simulink model "mech_robot"  (Simulink 6.0)
settings: Solver=ode15s  StartTime=0.0  StopTime=1  RelTol=1e-3  AbsTol=1e-4
PreLoadFcn:
  | load mech_robot_images;mech_robot_data;
undefined symbols (not defined in the file or in its folder): Actuator, rad, s
libraries: mblibv1 x88, mech_robot_vrlib x1
(part 1 of 3)
settings Model: Creator=gwood  LastModifiedBy=batserve  ExtModeAutoUpdateStatusClock=off  ProdHWDeviceType=Specified
settings DataIOCC: SignalLoggingName=sigsOut  OutputTimes=0:0.02:1
settings DebuggingCC: AlgebraicLoopMsg=none  CheckExecutionContextPreStartOutputMsg=on  CheckExecutionContextRuntimeOutputMsg=on  SolverPrmCheckMsg=none  UnconnectedInputMsg=none  UnconnectedOutputMsg=none  UnconnectedLineMsg=none
settings HardwareCC: ProdBitPerShort=32  ProdBitPerInt=16  ProdHWDeviceType=Specified  TargetUnknown=on

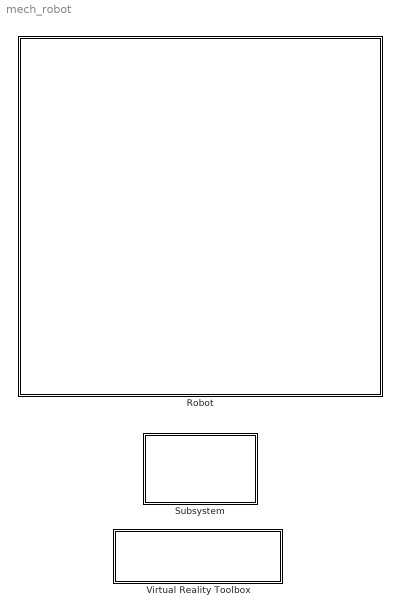
== system mech_robot ==
  Robot : Subsystem
      mask Display: image(robot);
  Subsystem : Subsystem
      mask Display: disp('Model Information');
  Virtual Reality Toolbox : Subsystem
      settings: AttributesFormatString=\n  OpenFcn=mech_OpenVrWorld(gcs,'mech_robot_vrlib')
      mask Type: Double-click open
      mask Display: disp(sprintf('Double-click to open\nVirtual Reality Toolbox viewer'))

== system mech_robot/Robot ==
  Joint Angles : Scope
  Link 1 : Subsystem  Orientation=up
      mask Display: image(rbody1)
  Link 2 : Subsystem
      mask Display: image(rbody2);
  Link3 : Subsystem  Orientation=up
      mask Display: image(rbody3);
  Link4 : Subsystem  Orientation=up
      mask Display: image(rbody4);
  Link5 : Subsystem  Orientation=up
      mask Display: image(rbody5);
  Link6 : Subsystem  Orientation=up
      mask Display: image(rdrill);
  Mux : Mux  Inputs=6
  Robot base : Subsystem  Orientation=up
      mask Display: image(rbase);
  wires:
  [Body1] -> Mux/1
  [Body2] -> Mux/2
  [Body3] -> Mux/3
  [Body4] -> Mux/4
  [Body5] -> Mux/5
  [Body6] -> Mux/6
  Mux/1 -> Joint Angles/1
  connections:
  Robot base/RConn1 -- Link 1/LConn1
  Link 1/RConn1 -- Link 2/LConn1
  Link 2/RConn1 -- Link3/LConn1
  Link3/RConn1 -- Link4/LConn1
  Link4/RConn1 -- Link5/LConn1
  Link5/RConn1 -- Link6/LConn1

== system mech_robot/Subsystem ==
  note: This model is a detailed dynamic model of the Siemens Manutec r3 robot. All of the important physical effects are
      | included, notably: the multibody dynamics, Coulomb friction, elasticity and damping in the gearboxes, the dynamics
      | of the motors including the current controller and the tachogenerators, and the cascade controllers. All of the parameters
      | of this model were obtained by experiment and can be found in the following paper. This model is used as a demanding
      | benchmark to test the simulation capabilites of robot simulation packages.
  note: "The Manutec r3 Benchmark Models for Dynamic Simulation of Robots", DLR FF-DR-ER, Technical Report TR T101-93,
      | March 1993.
  note: Paper available at: www.citeseer.com

== system mech_robot/Virtual Reality Toolbox ==
  VRAnimation : mech_robot_vrlib/mech_robot_arm_vr

== system mech_robot/Robot/Link 1 ==
  Body1 : mblibv1/Bodies/Body  Tag=Factory generic  Description=Mechanical Blockset  Orientation=up  PhysicalDomain=mechanical  SubClassName=Unknown  LeftPortType=workingframe  RightPortType=workingframe  LConnTagsString=CS1  RConnTagsString=CS2  DialogClass=MechanicalBodyBlock  Mass=0  MassUnits=kg  InertiaUnits=kg*m^2  Inertia=diag([0 1.16 0])  Shape=Cylinder  ShapeDims=[1 1]  ShapeUnits=m  ShapeUse=false  Density=1  DensityUnits=kg/m^3  DensityUse=false  CG=Left$CG$[0 -0.1750+0.25/2 0]$WORLD$WORLD$m$[0 0 0]$Euler X-Y-Z$deg$WORLD$false  WorkingFrames=Left$CS1$[0 -0.1750 0]$WORLD$WORLD$m$[0 0 0]$Euler X-Y-Z$deg$WORLD$true#Right$CS2$[0.075 0 0]$WORLD$WORLD$m$[0 0 0]$Euler X-Y-Z$deg$WORLD$true#Right$CS3$[-0.075 -0.1750 0.1]$CG$CG$m$[0 0 0]$Euler X-Y-Z$deg$WORLD$false#Right$CS4$[0.075 -0.1750 0.1]$CG$CG$m$[0 0 0]$Euler X-Y-Z$deg$WORLD$false#Right$CS5$[0.075 -0.1750 -0.1]$CG$CG$m$[0 0 0]$Euler X-Y-Z$deg$WORLD$false#Right$CS6$[-0.075 -0.1750 -0.1]$CG$CG$m$[0 0 0]$Euler X-Y-Z$deg$WORLD$false#Right$CS7$[-0.075 0.075 0.1]$CG$CG$m$[0 0 0]$Euler X-Y-Z$deg$WORLD$false#Right$CS8$[0.075 0.075 0.1]$CG$CG$m$[0 0 0]$Euler X-Y-Z$deg$WORLD$false#Right$CS9$[0.075 0.075 -0.1]$CG$CG$m$[0 0 0]$Euler X-Y-Z$deg$WORLD$false#Right$CS10$[-0.075 0.075 -0.1]$CG$CG$m$[0 0 0]$Euler X-Y-Z$deg$WORLD$false
  Drive1 : Subsystem  Orientation=up  mask{q0=-1, Actuator=Actuator{1}}
      mask prompts: q0 "Initial angle (rad)"; Actuator "Actuator data structure"
      settings: AttributesFormatString=\n
      mask Display: plot(-80,-80,80,80,[0,9,18,24,29,30,29,24,18,9,0,-9,-18,-24,-29,-30,-29,-24,-18,-9,0],[30,29,24,18,9,0,-9,-18,-24,-29,-30,-29,-24,-18,-9,0,9,18,24,29,30],[-29,-35,-35,-29],[-8,-8,8,8],[29,35,35,29],[-8,-8,8,8],[-35,-55],[0,0],[35,55],[0,0],[-78,-50,-50,-49,-45,-39,-33,-26,-21,-18,-17,-19,-22,-22,-26,-27,-25,-22,-16,-9,-3,2,6,6,4,1,1,-3,-4,-2,2,7,14,20,26,29,30,28,24,24,21,20,21,25,31,37,44,49,50,50,50,78]*.7,[58,58,57.2,49.2,42.8,38.8,38,39.6,44.4,51.6,59.6,67.6,72.4,72.4,65.2,57.2,49.2,42.8,38.8,38,39.6,44.4,51.6,59.6,67.6,72.4,72.4,65.2,57.2,49.2,42.8,38.8,38,39.6,44.4,51.6,59.6,67.6,72.4,72.4,65.2,57.2,49.2,42.8,38.8,38,39.6,44.4,51.6,58,58,58]*.6+15 );
  Trajectory 1 : Subsystem
  Follower : PMIOPort  Orientation=down  Port=1  Side=Right
  Base : PMIOPort  Orientation=up  Port=2  Side=Left
  wires:
  Trajectory 1/1(Acceleration1) -> Drive1/1(Acceleration)
  connections:
  Drive1/RConn1 -- Body1/LConn1
  Follower/RConn1 -- Body1/RConn1
  Base/RConn1 -- Drive1/LConn1

== system mech_robot/Robot/Link 2 ==
  Body2 : mblibv1/Bodies/Body  Tag=Factory generic  Description=Mechanical Blockset  Orientation=up  PhysicalDomain=mechanical  SubClassName=Unknown  LeftPortType=workingframe  RightPortType=workingframe  LConnTagsString=CS1  RConnTagsString=CS2  DialogClass=MechanicalBodyBlock  Mass=56.5  MassUnits=kg  InertiaUnits=kg*m^2  Inertia=[2.58 -0.46 0;-0.46 0.64 0;0 0 2.73]  Shape=Cylinder  ShapeDims=[1 1]  ShapeUnits=m  ShapeUse=false  Density=1  DensityUnits=kg/m^3  DensityUse=false  CG=Left$CG$[0.172 0.205 0]$WORLD$WORLD$m$[0 0 0]$Euler X-Y-Z$deg$WORLD$false  WorkingFrames=Left$CS1$[0.075 0 0]$WORLD$WORLD$m$[0 0 0]$Euler X-Y-Z$deg$WORLD$true#Right$CS2$[0.075 0.5 0]$WORLD$WORLD$m$[0 0 0]$Euler X-Y-Z$deg$WORLD$true#Right$CS3$[0.075 -0.1 0.1]$WORLD$WORLD$m$[0 0 0]$Euler X-Y-Z$deg$WORLD$false#Right$CS4$[0.075 0.6 0.1]$WORLD$WORLD$m$[0 0 0]$Euler X-Y-Z$deg$WORLD$false#Right$CS5$[0.075 0.6 -0.1]$WORLD$WORLD$m$[0 0 0]$Euler X-Y-Z$deg$WORLD$false#Right$CS6$[0.075 -0.1 -0.1]$WORLD$WORLD$m$[0 0 0]$Euler X-Y-Z$deg$WORLD$false#Right$CS7$[0.225 -0.1 -0.1]$WORLD$WORLD$m$[0 0 0]$Euler X-Y-Z$deg$WORLD$false#Right$CS8$[0.225 -0.1 0.1]$WORLD$WORLD$m$[0 0 0]$Euler X-Y-Z$deg$WORLD$false#Right$CS9$[0.225 0.6 0.1]$WORLD$WORLD$m$[0 0 0]$Euler X-Y-Z$deg$WORLD$false#Right$CS10$[0.225 0.6 -0.1]$WORLD$WORLD$m$[0 0 0]$Euler X-Y-Z$deg$WORLD$false
  Drive2 : Subsystem  Orientation=up  mask{q0=0.43, Actuator=Actuator{2}}
      mask prompts: q0 "Initial angle (rad)"; Actuator "Actuator data structure"
      mask Display: plot(-80,-80,80,80,[0,9,18,24,29,30,29,24,18,9,0,-9,-18,-24,-29,-30,-29,-24,-18,-9,0],[30,29,24,18,9,0,-9,-18,-24,-29,-30,-29,-24,-18,-9,0,9,18,24,29,30],[-29,-35,-35,-29],[-8,-8,8,8],[29,35,35,29],[-8,-8,8,8],[-35,-55],[0,0],[35,55],[0,0],[-78,-50,-50,-49,-45,-39,-33,-26,-21,-18,-17,-19,-22,-22,-26,-27,-25,-22,-16,-9,-3,2,6,6,4,1,1,-3,-4,-2,2,7,14,20,26,29,30,28,24,24,21,20,21,25,31,37,44,49,50,50,50,78]*.7,[58,58,57.2,49.2,42.8,38.8,38,39.6,44.4,51.6,59.6,67.6,72.4,72.4,65.2,57.2,49.2,42.8,38.8,38,39.6,44.4,51.6,59.6,67.6,72.4,72.4,65.2,57.2,49.2,42.8,38.8,38,39.6,44.4,51.6,59.6,67.6,72.4,72.4,65.2,57.2,49.2,42.8,38.8,38,39.6,44.4,51.6,58,58,58]*.6+15 );
  Subsystem : Subsystem
  Follower : PMIOPort  Orientation=down  Port=1  Side=Right
  Base : PMIOPort  Orientation=up  Port=2  Side=Left
  wires:
  Subsystem/1(Acceleration2) -> Drive2/1(Acceleration)
  connections:
  Follower/RConn1 -- Body2/RConn1
  Base/RConn1 -- Drive2/LConn1
  Drive2/RConn1 -- Body2/LConn1

== system mech_robot/Robot/Link3 ==
  Acceleration3 : Subsystem
  Body3 : mblibv1/Bodies/Body  Tag=Factory generic  Description=Mechanical Blockset  Orientation=up  PhysicalDomain=mechanical  SubClassName=Unknown  LeftPortType=workingframe  RightPortType=workingframe  LConnTagsString=CS1  RConnTagsString=CS2  DialogClass=MechanicalBodyBlock  Mass=26.4  MassUnits=kg  InertiaUnits=kg*m^2  Inertia="[0.279  -0.070  0;-0.070  0.245  0;0  0   0.413]"  Shape=Cylinder  ShapeDims=[1 1]  ShapeUnits=m  ShapeUse=false  Density=1  DensityUnits=kg/m^3  DensityUse=false  CG=Left$CG$[0.064 0.5-0.034 0]$WORLD$WORLD$m$[0 0 0]$Euler X-Y-Z$deg$WORLD$false  WorkingFrames=Left$CS1$[0.075 0.5 0]$WORLD$WORLD$m$[0 0 0]$Euler X-Y-Z$deg$WORLD$true#Right$CS2$[0 0.5+0.075 0]$WORLD$WORLD$m$[0 0 0]$Euler X-Y-Z$deg$WORLD$true#Right$CS3$[-0.075 0.5-0.075 0.075]$WORLD$WORLD$m$[0 0 0]$Euler X-Y-Z$deg$WORLD$false#Right$CS4$[0.075 0.5-0.075 0.075]$WORLD$WORLD$m$[0 0 0]$Euler X-Y-Z$deg$WORLD$false#Right$CS5$[0.075 0.5-0.075 -0.075]$WORLD$WORLD$m$[0 0 0]$Euler X-Y-Z$deg$WORLD$false#Right$CS6$[-0.075 0.5-0.075 -0.075]$WORLD$WORLD$m$[0 0 0]$Euler X-Y-Z$deg$WORLD$false#Right$CS7$[-0.075 0.5+0.075 0.075]$WORLD$WORLD$m$[0 0 0]$Euler X-Y-Z$deg$WORLD$false#Right$CS8$[-0.075 0.5+0.075 -0.075]$WORLD$WORLD$m$[0 0 0]$Euler X-Y-Z$deg$WORLD$false#Right$CS9$[0.075 0.5+0.075 -0.075]$WORLD$WORLD$m$[0 0 0]$Euler X-Y-Z$deg$WORLD$false#Right$CS10$[0.075 0.5+0.075 0.075]$WORLD$WORLD$m$[0 0 0]$Euler X-Y-Z$deg$WORLD$false
  Drive3 : Subsystem  Orientation=up  mask{q0=1.57, Actuator=Actuator{3}}
      mask prompts: q0 "Initial angle (rad)"; Actuator "Actuator data structure"
      mask Display: plot(-80,-80,80,80,[0,9,18,24,29,30,29,24,18,9,0,-9,-18,-24,-29,-30,-29,-24,-18,-9,0],[30,29,24,18,9,0,-9,-18,-24,-29,-30,-29,-24,-18,-9,0,9,18,24,29,30],[-29,-35,-35,-29],[-8,-8,8,8],[29,35,35,29],[-8,-8,8,8],[-35,-55],[0,0],[35,55],[0,0],[-78,-50,-50,-49,-45,-39,-33,-26,-21,-18,-17,-19,-22,-22,-26,-27,-25,-22,-16,-9,-3,2,6,6,4,1,1,-3,-4,-2,2,7,14,20,26,29,30,28,24,24,21,20,21,25,31,37,44,49,50,50,50,78]*.7,[58,58,57.2,49.2,42.8,38.8,38,39.6,44.4,51.6,59.6,67.6,72.4,72.4,65.2,57.2,49.2,42.8,38.8,38,39.6,44.4,51.6,59.6,67.6,72.4,72.4,65.2,57.2,49.2,42.8,38.8,38,39.6,44.4,51.6,59.6,67.6,72.4,72.4,65.2,57.2,49.2,42.8,38.8,38,39.6,44.4,51.6,58,58,58]*.6+15 );
  Follower : PMIOPort  Orientation=down  Port=1  Side=Right
  Base : PMIOPort  Orientation=up  Port=2  Side=Left
  wires:
  Acceleration3/1(Acceleration3) -> Drive3/1(Acceleration)
  connections:
  Drive3/RConn1 -- Body3/LConn1
  Follower/RConn1 -- Body3/RConn1
  Base/RConn1 -- Drive3/LConn1

== system mech_robot/Robot/Link4 ==
  Body4 : mblibv1/Bodies/Body  Tag=Factory generic  Description=Mechanical Blockset  Orientation=up  PhysicalDomain=mechanical  SubClassName=Unknown  LeftPortType=workingframe  RightPortType=workingframe  LConnTagsString=CS1  RConnTagsString=CS2  DialogClass=MechanicalBodyBlock  Mass=28.7  MassUnits=kg  InertiaUnits=kg*m^2  Inertia=[1.67 0 0;0 0.081 0;0 0 1.67]  Shape=Cylinder  ShapeDims=[1 1]  ShapeUnits=m  ShapeUse=false  Density=1  DensityUnits=kg/m^3  DensityUse=false  CG=Left$CG$[0 0.5+0.32 0]$WORLD$WORLD$m$[0 0 0]$Euler X-Y-Z$deg$WORLD$false  WorkingFrames=Left$CS1$[0 0.5+0.075 0]$WORLD$WORLD$m$[0 0 0]$Euler X-Y-Z$deg$WORLD$true#Right$CS2$[0 0.5+0.73 0]$WORLD$WORLD$m$[0 0 0]$Euler X-Y-Z$deg$WORLD$true#Right$CS3$[-0.05 0.5+0.075 -0.05]$WORLD$WORLD$m$[0 0 0]$Euler X-Y-Z$deg$WORLD$false#Right$CS4$[0.05 0.5+0.075 -0.05]$WORLD$WORLD$m$[0 0 0]$Euler X-Y-Z$deg$WORLD$false#Right$CS5$[0.05 0.5+0.075 0.05]$WORLD$WORLD$m$[0 0 0]$Euler X-Y-Z$deg$WORLD$false#Right$CS6$[-0.05 0.5+0.075 0.05]$WORLD$WORLD$m$[0 0 0]$Euler X-Y-Z$deg$WORLD$false#Right$CS7$[0.05 0.5+0.075+0.73 -0.05]$WORLD$WORLD$m$[0 0 0]$Euler X-Y-Z$deg$WORLD$false#Right$CS8$[-0.05 0.5+0.075+0.73 0.05]$WORLD$WORLD$m$[0 0 0]$Euler X-Y-Z$deg$WORLD$false#Right$CS9$[-0.05 0.5+0.075+0.73 -0.05]$WORLD$WORLD$m$[0 0 0]$Euler X-Y-Z$deg$WORLD$false#Right$CS10$[0.05 0.5+0.075+0.73 0.05]$WORLD$WORLD$m$[0 0 0]$Euler X-Y-Z$deg$WORLD$false
  Drive4 : Subsystem  Orientation=up  mask{q0=0, Actuator=Actuator{4}}
      mask prompts: q0 "Initial rotation (rad)"; Actuator "Actuator data structure"
      mask Display: plot(-80,-80,80,80,[0,9,18,24,29,30,29,24,18,9,0,-9,-18,-24,-29,-30,-29,-24,-18,-9,0],[30,29,24,18,9,0,-9,-18,-24,-29,-30,-29,-24,-18,-9,0,9,18,24,29,30],[-29,-35,-35,-29],[-8,-8,8,8],[29,35,35,29],[-8,-8,8,8],[-35,-55],[0,0],[35,55],[0,0],[-78,-50,-50,-49,-45,-39,-33,-26,-21,-18,-17,-19,-22,-22,-26,-27,-25,-22,-16,-9,-3,2,6,6,4,1,1,-3,-4,-2,2,7,14,20,26,29,30,28,24,24,21,20,21,25,31,37,44,49,50,50,50,78]*.7,[58,58,57.2,49.2,42.8,38.8,38,39.6,44.4,51.6,59.6,67.6,72.4,72.4,65.2,57.2,49.2,42.8,38.8,38,39.6,44.4,51.6,59.6,67.6,72.4,72.4,65.2,57.2,49.2,42.8,38.8,38,39.6,44.4,51.6,59.6,67.6,72.4,72.4,65.2,57.2,49.2,42.8,38.8,38,39.6,44.4,51.6,58,58,58]*.6+15 );
  Subsystem1 : Subsystem
  Follower : PMIOPort  Orientation=down  Port=1  Side=Right
  Base : PMIOPort  Orientation=up  Port=2  Side=Left
  wires:
  Subsystem1/1(Acceleration4) -> Drive4/1(Acceleration)
  connections:
  Drive4/RConn1 -- Body4/LConn1
  Follower/RConn1 -- Body4/RConn1
  Base/RConn1 -- Drive4/LConn1

== system mech_robot/Robot/Link5 ==
  Body5 : mblibv1/Bodies/Body  Tag=Factory generic  Description=Mechanical Blockset  Orientation=up  PhysicalDomain=mechanical  SubClassName=Unknown  LeftPortType=workingframe  RightPortType=workingframe  LConnTagsString=CS1  RConnTagsString=CS2  DialogClass=MechanicalBodyBlock  Mass=5.2  MassUnits=kg  InertiaUnits=kg*m^2  Inertia=[1.25 0 0;0 0.81 0;0 0 1.53]  Shape=Cylinder  ShapeDims=[1 1]  ShapeUnits=m  ShapeUse=false  Density=1  DensityUnits=kg/m^3  DensityUse=false  CG=Left$CG$[0 0.5+0.73+0.023 0]$WORLD$WORLD$m$[0 0 0]$Euler X-Y-Z$deg$WORLD$false  WorkingFrames=Left$CS1$[0 0.5+0.73 0]$WORLD$WORLD$m$[0 0 0]$Euler X-Y-Z$deg$WORLD$true#Right$CS2$[0 0.5+0.73 0]$WORLD$WORLD$m$[0 0 0]$Euler X-Y-Z$deg$WORLD$true#Left$CS3$[-0.0375 0.5+0.73 0.05]$WORLD$WORLD$m$[0 0 0]$Euler X-Y-Z$deg$WORLD$false#Left$CS4$[-0.0375 0.5+0.73 -0.05]$WORLD$WORLD$m$[0 0 0]$Euler X-Y-Z$deg$WORLD$false#Left$CS5$[0.0375 0.5+0.73 -0.05]$WORLD$WORLD$m$[0 0 0]$Euler X-Y-Z$deg$WORLD$false#Left$CS6$[0.0375 0.5+0.73 0.05]$WORLD$WORLD$m$[0 0 0]$Euler X-Y-Z$deg$WORLD$false#Left$CS7$[0.0375 0.5+0.73+0.225 -0.05]$WORLD$WORLD$m$[0 0 0]$Euler X-Y-Z$deg$WORLD$false#Left$CS9$[0.0375 0.5+0.73+0.225 0.05]$WORLD$WORLD$m$[0 0 0]$Euler X-Y-Z$deg$WORLD$false#Left$CS8$[-0.0375 0.5+0.73+0.225 0.05]$WORLD$WORLD$m$[0 0 0]$Euler X-Y-Z$deg$WORLD$false#Left$CS10$[-0.0375 0.5+0.73+0.225 -0.05]$WORLD$WORLD$m$[0 0 0]$Euler X-Y-Z$deg$WORLD$false
  Drive5 : Subsystem  Orientation=up  mask{q0=-2, Actuator=Actuator{5}}
      mask prompts: q0 "Initial rotation (rad)"; Actuator "Actuator data structure"
      mask Display: plot(-80,-80,80,80,[0,9,18,24,29,30,29,24,18,9,0,-9,-18,-24,-29,-30,-29,-24,-18,-9,0],[30,29,24,18,9,0,-9,-18,-24,-29,-30,-29,-24,-18,-9,0,9,18,24,29,30],[-29,-35,-35,-29],[-8,-8,8,8],[29,35,35,29],[-8,-8,8,8],[-35,-55],[0,0],[35,55],[0,0],[-78,-50,-50,-49,-45,-39,-33,-26,-21,-18,-17,-19,-22,-22,-26,-27,-25,-22,-16,-9,-3,2,6,6,4,1,1,-3,-4,-2,2,7,14,20,26,29,30,28,24,24,21,20,21,25,31,37,44,49,50,50,50,78]*.7,[58,58,57.2,49.2,42.8,38.8,38,39.6,44.4,51.6,59.6,67.6,72.4,72.4,65.2,57.2,49.2,42.8,38.8,38,39.6,44.4,51.6,59.6,67.6,72.4,72.4,65.2,57.2,49.2,42.8,38.8,38,39.6,44.4,51.6,59.6,67.6,72.4,72.4,65.2,57.2,49.2,42.8,38.8,38,39.6,44.4,51.6,58,58,58]*.6+15 );
  Subsystem2 : Subsystem
  Follower : PMIOPort  Orientation=down  Port=1  Side=Right
  Base : PMIOPort  Orientation=up  Port=2  Side=Left
  wires:
  Subsystem2/1(Acceleration5) -> Drive5/1(Acceleration)
  connections:
  Drive5/RConn1 -- Body5/LConn1
  Follower/RConn1 -- Body5/RConn1
  Base/RConn1 -- Drive5/LConn1

== system mech_robot/Robot/Link6 ==
  Body6 : mblibv1/Bodies/Body  Tag=Factory generic  Description=Mechanical Blockset  Orientation=up  PhysicalDomain=mechanical  SubClassName=Unknown  LeftPortType=workingframe  RightPortType=workingframe  LConnTagsString=CS1  DialogClass=MechanicalBodyBlock  Mass=2.4063  MassUnits=kg  InertiaUnits=kg*m^2  Inertia="2.4063/12*diag([0.125^2+0.05^2  0.05^2+0.05^2  0.125^2+0.05^2])"  Shape=Cylinder  ShapeDims=[1 1]  ShapeUnits=m  ShapeUse=false  Density=1  DensityUnits=kg/m^3  DensityUse=false  CG=Left$CG$[0 0.5+0.73+0.15+0.125/2 0]$WORLD$WORLD$m$[0 0 0]$Euler X-Y-Z$deg$WORLD$false  WorkingFrames=Left$CS1$[0 0.5+0.73 0]$WORLD$WORLD$m$[0 0 0]$Euler X-Y-Z$deg$WORLD$true#Left$CS2$[-0.025 0.5+0.73+0.15 0.025]$WORLD$WORLD$m$[0 0 0]$Euler X-Y-Z$deg$WORLD$false#Left$CS3$[-0.025 0.5+0.73+0.15 -0.025]$WORLD$WORLD$m$[0 0 0]$Euler X-Y-Z$deg$WORLD$false#Left$CS4$[0.025 0.5+0.73+0.15 -0.025]$WORLD$WORLD$m$[0 0 0]$Euler X-Y-Z$deg$WORLD$false#Left$CS5$[0.025 0.5+0.73+0.15 0.025]$WORLD$WORLD$m$[0 0 0]$Euler X-Y-Z$deg$WORLD$false#Left$CS6$[0.025 0.5+0.73+0.15+0.125 0.025]$WORLD$WORLD$m$[0 0 0]$Euler X-Y-Z$deg$WORLD$false#Left$CS7$[0.025 0.5+0.73+0.15+0.125 -0.025]$WORLD$WORLD$m$[0 0 0]$Euler X-Y-Z$deg$WORLD$false#Left$CS8$[-0.025 0.5+0.73+0.15+0.125 -0.025]$WORLD$WORLD$m$[0 0 0]$Euler X-Y-Z$deg$WORLD$false#Left$CS9$[-0.025 0.5+0.73+0.15+0.125 0.025]$WORLD$WORLD$m$[0 0 0]$Euler X-Y-Z$deg$WORLD$false
  Drive6 : Subsystem  Orientation=up  mask{q0=0, Actuator=Actuator{6}}
      mask prompts: q0 "Initial rotation (rad)"; Actuator "Actuator data structure"
      mask Display: plot(-80,-80,80,80,[0,9,18,24,29,30,29,24,18,9,0,-9,-18,-24,-29,-30,-29,-24,-18,-9,0],[30,29,24,18,9,0,-9,-18,-24,-29,-30,-29,-24,-18,-9,0,9,18,24,29,30],[-29,-35,-35,-29],[-8,-8,8,8],[29,35,35,29],[-8,-8,8,8],[-35,-55],[0,0],[35,55],[0,0],[-78,-50,-50,-49,-45,-39,-33,-26,-21,-18,-17,-19,-22,-22,-26,-27,-25,-22,-16,-9,-3,2,6,6,4,1,1,-3,-4,-2,2,7,14,20,26,29,30,28,24,24,21,20,21,25,31,37,44,49,50,50,50,78]*.7,[58,58,57.2,49.2,42.8,38.8,38,39.6,44.4,51.6,59.6,67.6,72.4,72.4,65.2,57.2,49.2,42.8,38.8,38,39.6,44.4,51.6,59.6,67.6,72.4,72.4,65.2,57.2,49.2,42.8,38.8,38,39.6,44.4,51.6,59.6,67.6,72.4,72.4,65.2,57.2,49.2,42.8,38.8,38,39.6,44.4,51.6,58,58,58]*.6+15 );
  Subsystem3 : Subsystem
  "Base " : PMIOPort  Orientation=up  Port=1  Side=Left
  wires:
  Subsystem3/1(Acceleration6) -> Drive6/1(Acceleration)
  connections:
  Drive6/RConn1 -- Body6/LConn1
  "Base "/RConn1 -- Drive6/LConn1

== system mech_robot/Robot/Robot base ==
  Body0 : mblibv1/Bodies/Body  Tag=Factory generic  Description=Mechanical Blockset  Orientation=up  PhysicalDomain=mechanical  SubClassName=Unknown  LeftPortType=workingframe  RightPortType=workingframe  LConnTagsString=CS1  RConnTagsString=CS2  DialogClass=MechanicalBodyBlock  Mass=1  MassUnits=kg  InertiaUnits=kg*m^2  Inertia=eye(3)  Shape=Cylinder  ShapeDims=[1 1]  ShapeUnits=m  ShapeUse=false  Density=1  DensityUnits=kg/m^3  DensityUse=false  CG=Left$CG$[0 -0.2875 0 ]$WORLD$WORLD$m$[0 0 0]$Euler X-Y-Z$deg$WORLD$false  WorkingFrames=Left$CS1$[0 -0.4 0]$WORLD$WORLD$m$[0 0 0]$Euler X-Y-Z$deg$WORLD$true#Right$CS2$[0 -0.1750 0]$WORLD$WORLD$m$[0 0 0]$Euler X-Y-Z$deg$WORLD$true#Right$CS3$[0.3 -0.4 -0.3]$WORLD$WORLD$m$[0 0 0]$Euler X-Y-Z$deg$WORLD$false#Right$CS4$[-0.3 -0.4 -0.3]$WORLD$WORLD$m$[0 0 0]$Euler X-Y-Z$deg$WORLD$false#Left$CS9$[-0.3 -0.4 0.3]$WORLD$WORLD$m$[0 0 0]$Euler X-Y-Z$deg$WORLD$false#Right$CS10$[0.3 -0.4 0.3]$WORLD$WORLD$m$[0 0 0]$Euler X-Y-Z$deg$WORLD$false#Right$CS5$[-0.3 -0.1750 -0.3]$WORLD$WORLD$m$[0 0 0]$Euler X-Y-Z$deg$WORLD$false#Right$CS6$[-0.3 -0.1750 0.3]$WORLD$WORLD$m$[0 0 0]$Euler X-Y-Z$deg$WORLD$false#Right$CS7$[0.3 -0.1750 0.3]$WORLD$WORLD$m$[0 0 0]$Euler X-Y-Z$deg$WORLD$false#Right$CS8$[0.3 -0.1750 -0.3]$WORLD$WORLD$m$[0 0 0]$Euler X-Y-Z$deg$WORLD$false
  Inertial Frame : mblibv1/Bodies/Ground  Orientation=up  Opaque=on  LeftPortType=env  RightPortType=workingframe  PhysicalDomain=Mechanical  DialogClass=GroundBlock  CoordPosition=[0 -0.4 0]  CoordPositionUnits=m  StateVectorMgrId=-1  MachineId=[0 0]  ShowEnvPort=on
  Machine Environment : mblibv1/Bodies/Machine Environment  Tag=Factory ground  Orientation=up  DialogController=MECH.DialogSource  Opaque=on  PortType=env  PhysicalDomain=Mechanical  DialogTemplateClass=MECH.MachineEnvironment  SyncWhenCopied=off  Gravity=[0 -9.81 0]  GravityUnits=m/s^2  GravityAsSignal=off  Dimensionality=3D Only  AnalysisType=Forward dynamics  LinearAssemblyTolerance=1e-3  LinearAssemblyToleranceUnits=m  AngularAssemblyTolerance=1e-3  AngularAssemblyToleranceUnits=rad  ConstraintSolverType=Stabilizing  ConstraintRelTolerance=1e-4  ConstraintAbsTolerance=1e-4  UseRobustSingularityHandling=off  StatePerturbationType=Fixed  PerturbationSize=1e-5  VisualizeMachine=on
  Weld : mblibv1/Joints/Weld  Tag=Factory generic  Description=Mechanical Blockset  Orientation=up  PhysicalDomain=mechanical  SubClassName=Unknown  LeftPortType=blob  RightPortType=blob  LConnTagsString=__newl0  RConnTagsString=__newr0  NumSAPorts=0  CutJoint=off  MarkAsCut=off  Primitives=weld  PrimitiveProps=W$INERTIAL$[0 0 0]$weld  DialogClass=JointBlock
  Follower : PMIOPort  Orientation=down  Port=1  Side=Right
  connections:
  Weld/RConn1 -- Body0/LConn1
  Inertial Frame/RConn1 -- Weld/LConn1
  Follower/RConn1 -- Body0/RConn1
  Machine Environment/RConn1 -- Inertial Frame/LConn1

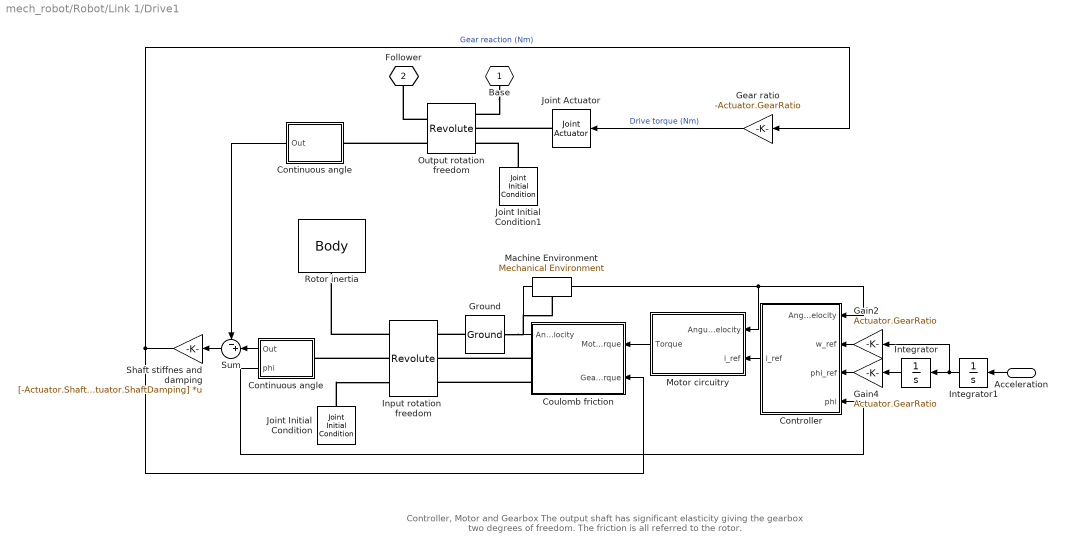
== system mech_robot/Robot/Link 1/Drive1 ==
  note: Controller, Motor and Gearbox
      |
      | The output shaft has significant elasticity giving the gearbox two
      | degrees of freedom. The friction is all referred to the rotor.
  Acceleration : Inport  Orientation=left  Port=1  LatchInput=off
  Continuous angle : Subsystem  Orientation=left
  "Continuous angle " : Subsystem  Orientation=left
  Controller : Subsystem  Orientation=left
  Coulomb friction : Subsystem  Orientation=left  mask{peak=Actuator.PeakRatio, Rv1=Actuator.FrictionGain, Rv0=Actuator.FrictionConstant}
      mask prompts: peak "Peak ratio"; Rv1 "Friction gain (Nm.s/rad)"; Rv0 "Friction constant (Nm)"
      mask Display:
      | plot([-2 0 0 2],[-2 -1 1 2]);
      | plot([-5 5],[0 0]);
      | plot([0 0],[-5 5]);
      | plot([-0.02 -0.02],[-3 3]);
      | plot([-0.04 -0.04],[-3 3]);
      | plot([-0.06 -0.06],[-3 3]);
      | plot([-0.08 -0.08],[-3 3]);
      | plot([-0.1 -0.1],[-3 3]);
      | plot([0.02 0.02],[-3 3]);
      | plot([0.04 0.04],[-3 3]);
      | plot([0.06 0.06],[-3 3]);
      | plot([0.08 0.08],[-3 3]);
      | plot([0.1 0.1],[-3 3]);
      | plot([-2 0],[-2.03 -1.03]);
      | plot([-2 0],[-2.06 -1.06]);
      | plot([-2 0],[-2.09 -1.09]);
      | plot([-2 0],[-2.12 -1.21]);
      | plot([-2 0],[-1.97 -0.97]);
      | plot([-2 0],[-1.94 -0.94]);
      | plot([-2 0],[-1.91 -0.91]);
      | plot([-2 0],[-1.88 -0.88]);
      | 
      | plot([2 0],[2.03 1.03]);
      | plot([2 0],[2.06 1.06]);
      | plot([2 0],[2.09 1.09]);
      | plot([2 0],[2.12 1.21]);
      | plot([2 0],[1.97 0.97]);
      | plot([2 0],[1.94 0.94]);
      | plot([2 0],[1.91 0.91]);
      | plot([2 0],[1.88 0.88]);
  Gain2 : Gain  Orientation=left  Gain=Actuator.GearRatio  SaturateOnIntegerOverflow=on
  Gain4 : Gain  Orientation=left  Gain=Actuator.GearRatio  SaturateOnIntegerOverflow=on
  Gear ratio : Gain  Orientation=left  Gain=-Actuator.GearRatio  SaturateOnIntegerOverflow=on
  Ground : mblibv1/Bodies/Ground  Orientation=left  Opaque=on  LeftPortType=env  RightPortType=workingframe  PhysicalDomain=Mechanical  DialogClass=GroundBlock  CoordPosition=[0 0 0]  CoordPositionUnits=m  StateVectorMgrId=-1  MachineId=[7 0]  ShowEnvPort=on
  Input rotation  freedom : mblibv1/Joints/Revolute  Tag=Factory generic  Description=Mechanical Blockset  Orientation=left  PhysicalDomain=mechanical  SubClassName=Unknown  LeftPortType=blob  RightPortType=blob  LConnTagsString=__newl0|SA1|SA2  RConnTagsString=__newr0|SA1|SA2  NumSAPorts=4  CutJoint=off  MarkAsCut=off  Primitives=revolute  PrimitiveProps=R1$WORLD$Actuator.Axis$revolute  DialogClass=JointBlock
  Integrator : Integrator  Orientation=left  InitialCondition=q0  ZeroCross=off
  Integrator1 : Integrator  Orientation=left  ZeroCross=off
  Joint Actuator : mblibv1/Sensors &  Actuators/Joint Actuator  Orientation=left  Opaque=on  PhysicalDomain=Mechanical  PortType=blob  ActuationStyle=Force  AngleUnits=deg  ArcVelocityUnits=deg/s  ArcAccelerationUnits=deg/s^2  CoordPositionUnits=m  VelocityUnits=m/s  AccelerationUnits=m/s^2  ForceUnits=N  TorqueUnits=N-m  ActiveIO=on  Width=1  DialogClass=MechanicalActuatorBlock  Primitive=R1  ReferenceFrame=Absolute (INERTIAL)
  Joint Initial Condition : mblibv1/Sensors &  Actuators/Joint Initial Condition  Orientation=up  Opaque=on  PhysicalDomain=Mechanical  DialogClass=InitialConditionBlock  Primitive=R1  CoordPosition=q0*Actuator.GearRatio  Velocity=0.0  AngleUnits=rad  ArcVelocityUnits=deg/s  CoordPositionUnits=m  VelocityUnits=m/s  InitialConditions=P1$false$0$m$rad$0$m/s$rad/s#P2$false$0$m$rad$0$m/s$rad/s#P3$false$0$m$rad$0$m/s$rad/s#R1$true$q0*Actuator.GearRatio$m$rad$0.0$m/s$deg/s#R2$false$0$m$rad$0$m/s$rad/s#R3$false$0$m$rad$0$m/s$rad/s#S$false$0$m$rad$0$m/s$rad/s
  Joint Initial Condition1 : mblibv1/Sensors &  Actuators/Joint Initial Condition  Orientation=up  Opaque=on  PhysicalDomain=Mechanical  DialogClass=InitialConditionBlock  Primitive=R1  CoordPosition=q0  Velocity=0.0  AngleUnits=rad  ArcVelocityUnits=deg/s  CoordPositionUnits=m  VelocityUnits=m/s  InitialConditions=P1$false$0$m$rad$0$m/s$rad/s#P2$false$0$m$rad$0$m/s$rad/s#P3$false$0$m$rad$0$m/s$rad/s#R1$true$q0$m$rad$0.0$m/s$deg/s#R2$false$0$m$rad$0$m/s$rad/s#R3$false$0$m$rad$0$m/s$rad/s#S$false$0$m$rad$0$m/s$rad/s
  Machine Environment : mblibv1/Bodies/Mechanical Environment  Tag=Factory ground  Orientation=down  DialogController=MECH.DialogSource  Opaque=on  PortType=env  PhysicalDomain=Mechanical  DialogTemplateClass=MECH.MachineEnvironment  SyncWhenCopied=off  Gravity=[0 -9.81 0]  GravityUnits=m/s^2  GravityAsSignal=off  Dimensionality=3D Only  AnalysisType=Forward dynamics  LinearAssemblyTolerance=1e-3  LinearAssemblyToleranceUnits=m  AngularAssemblyTolerance=1e-3  AngularAssemblyToleranceUnits=rad  ConstraintSolverType=Stabilizing  ConstraintRelTolerance=1e-4  ConstraintAbsTolerance=1e-4  UseRobustSingularityHandling=off  StatePerturbationType=Fixed  PerturbationSize=1e-5  VisualizeMachine=on
  Motor circuitry : Subsystem  Orientation=left  mask{Ri=10, Ra=250, Rd1=100, Rd2=100, Rd3=100, Rd4=100, Rp1=200, Rp2=50, k=Actuator.MotorGain, d=Actuator.MotorDamping, w=Actuator.MotorConstant}
      mask prompts: Ri "Ri (Ohms)"; Ra "Ra (Ohms)"; Rd1 "Rd1 (Ohms)"; Rd2 "Rd2 (Ohms)"; Rd3 "Rd3 (Ohms)"; Rd4 "Rd4 (Ohms)"; Rp1 "Rp1 (Ohms)"; Rp2 "Rp2 (Ohms)"; k "Motor gain (Nm/A)"; d "Motor damping"; w "Motor time constant"
      mask Display: plot(-140,-140,140,140,2*[-30,-30,0,-30,-30,-55]+25,(2*[20,0,20,41,20,20]+8),[0,0]+25,(2*[0,40]+8),2*[37.5,0]+25,(2*[20,20]+8),2*[10,10,0]+25,(1*[-15,6,20]+12),1*[-65,-65,-20,-20,40,40,85,85,85,40,40,-20,-20],1*[48,-20,-20,-10,-10,-20,-20,48,-20,-20,-30,-30,-20])
  Output rotation freedom : mblibv1/Joints/Revolute  Tag=Factory generic  Description=Mechanical Blockset  Orientation=left  PhysicalDomain=mechanical  SubClassName=Unknown  LeftPortType=blob  RightPortType=blob  LConnTagsString=__newl0|SA1|SA2  RConnTagsString=__newr0|SA1  NumSAPorts=3  CutJoint=off  MarkAsCut=off  Primitives=revolute  PrimitiveProps=R1$WORLD$Actuator.Axis$revolute  DialogClass=JointBlock
  Rotor inertia : mblibv1/Bodies/Body  Tag=Factory generic  Description=Mechanical Blockset  Orientation=up  PhysicalDomain=mechanical  SubClassName=Unknown  LeftPortType=workingframe  RightPortType=workingframe  LConnTagsString=CS1  DialogClass=MechanicalBodyBlock  Mass=0  MassUnits=kg  InertiaUnits=kg*m^2  Inertia=Actuator.MotorInertia*eye(3)  Shape=Cylinder  ShapeDims=[1 1]  ShapeUnits=m  ShapeUse=false  Density=1  DensityUnits=kg/m^3  DensityUse=false  CG=Left$CG$[0 0 0]$CS1$CS1$m$[0 0 0]$Euler X-Y-Z$deg$WORLD$false  WorkingFrames=Left$CS1$[0 0 0]$ADJOINING$ADJOINING$m$[0 0 0]$Euler X-Y-Z$deg$WORLD$true
  Shaft stiffnes and damping : Gain  Orientation=left  Gain=[-Actuator.ShaftStiffness -Actuator.ShaftDamping]  Multiplication=Matrix(K*u)  SaturateOnIntegerOverflow=on
  Sum : Sum  Orientation=left  Inputs=-+|  SaturateOnIntegerOverflow=on  InputSameDT=on
  Base : PMIOPort  Tag=PMCPort  Orientation=down  Port=1  Side=Left
  Follower : PMIOPort  Tag=PMCPort  Orientation=down  Port=2  Side=Right
  wires:
  Coulomb friction/1(Angular velocity) -> Controller/1(Angular velocity), Motor circuitry/1(Angular velocity)
  Gear ratio/1 -> Joint Actuator/1  "Drive torque (Nm)"
  Integrator/1 -> Gain4/1
  Acceleration/1 -> Integrator1/1
  "Continuous angle "/1("Out ") -> Sum/1
  Gain2/1 -> Controller/2(w_ref)
  Gain4/1 -> Controller/3(phi_ref)
  Motor circuitry/1(Torque) -> Coulomb friction/1(Motor torque)
  Sum/1 -> Shaft stiffnes and damping/1
  Continuous angle/1(Out) -> Sum/2
  Continuous angle/2(phi) -> Controller/4(phi)
  Integrator1/1 -> Integrator/1, Gain2/1
  Shaft stiffnes and damping/1 -> Gear ratio/1, Coulomb friction/2(Gear torque)  "Gear reaction (Nm)"
  Controller/1(i_ref) -> Motor circuitry/2(i_ref)
  connections:
  Base/RConn1 -- Output rotation freedom/LConn1
  Output rotation freedom/RConn1 -- Follower/RConn1
  Output rotation freedom/RConn2 -- "Continuous angle "/LConn1
  Coulomb friction/RConn1 -- Input rotation  freedom/LConn2
  Coulomb friction/RConn2 -- Input rotation  freedom/LConn3
  Input rotation  freedom/RConn1 -- Rotor inertia/LConn1
  Input rotation  freedom/RConn2 -- Continuous angle/LConn1
  Ground/RConn1 -- Input rotation  freedom/LConn1
  Joint Initial Condition1/RConn1 -- Output rotation freedom/LConn3
  Joint Actuator/RConn1 -- Output rotation freedom/LConn2
  Joint Initial Condition/RConn1 -- Input rotation  freedom/RConn3
  Ground/LConn1 -- Machine Environment/RConn1

== system mech_robot/Robot/Link 1/Trajectory 1 ==
  Clock : Clock
      settings: Decimation=10
  Trajectory 1 : Lookup  DialogController=Simulink.DDGSource  InputValues="[0    0.1000    0.1000    0.7400    0.7400    1.1200    1.1200    1.2000    1.2000    1.3000]"  OutputValues="[30.0000   30.0000         0         0  -13.9600  -13.9600   28.7500   28.7500         0         0]"  SaturateOnIntegerOverflow=on
  Acceleration1 : Outport
  wires:
  Clock/1 -> Trajectory 1/1
  Trajectory 1/1 -> Acceleration1/1

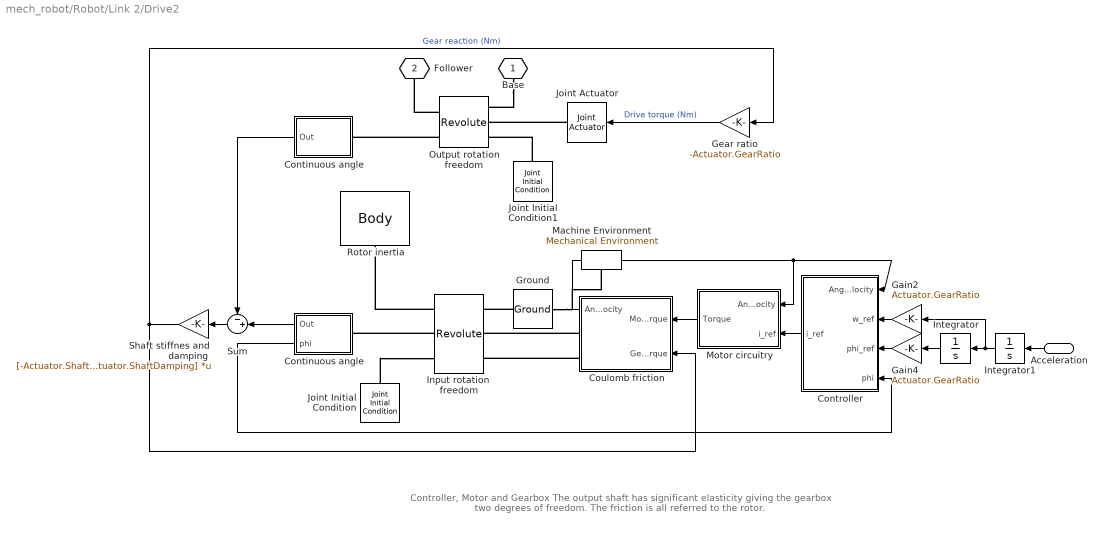
== system mech_robot/Robot/Link 2/Drive2 ==
  note: Controller, Motor and Gearbox
      |
      | The output shaft has significant elasticity giving the gearbox two
      | degrees of freedom. The friction is all referred to the rotor.
  Acceleration : Inport  Orientation=left  Port=1  LatchInput=off
  Continuous angle : Subsystem  Orientation=left
  "Continuous angle " : Subsystem  Orientation=left
  Controller : Subsystem  Orientation=left
  Coulomb friction : Subsystem  Orientation=left  mask{peak=Actuator.PeakRatio, Rv1=Actuator.FrictionGain, Rv0=Actuator.FrictionConstant}
      mask prompts: peak "Peak ratio"; Rv1 "Friction gain (Nm.s/rad)"; Rv0 "Friction constant (Nm)"
      mask Display:
      | plot([-2 0 0 2],[-2 -1 1 2]);
      | plot([-5 5],[0 0]);
      | plot([0 0],[-5 5]);
      | plot([-0.02 -0.02],[-3 3]);
      | plot([-0.04 -0.04],[-3 3]);
      | plot([-0.06 -0.06],[-3 3]);
      | plot([-0.08 -0.08],[-3 3]);
      | plot([-0.1 -0.1],[-3 3]);
      | plot([0.02 0.02],[-3 3]);
      | plot([0.04 0.04],[-3 3]);
      | plot([0.06 0.06],[-3 3]);
      | plot([0.08 0.08],[-3 3]);
      | plot([0.1 0.1],[-3 3]);
      | plot([-2 0],[-2.03 -1.03]);
      | plot([-2 0],[-2.06 -1.06]);
      | plot([-2 0],[-2.09 -1.09]);
      | plot([-2 0],[-2.12 -1.21]);
      | plot([-2 0],[-1.97 -0.97]);
      | plot([-2 0],[-1.94 -0.94]);
      | plot([-2 0],[-1.91 -0.91]);
      | plot([-2 0],[-1.88 -0.88]);
      | 
      | plot([2 0],[2.03 1.03]);
      | plot([2 0],[2.06 1.06]);
      | plot([2 0],[2.09 1.09]);
      | plot([2 0],[2.12 1.21]);
      | plot([2 0],[1.97 0.97]);
      | plot([2 0],[1.94 0.94]);
      | plot([2 0],[1.91 0.91]);
      | plot([2 0],[1.88 0.88]);
  Gain2 : Gain  Orientation=left  Gain=Actuator.GearRatio  SaturateOnIntegerOverflow=on
  Gain4 : Gain  Orientation=left  Gain=Actuator.GearRatio  SaturateOnIntegerOverflow=on
  Gear ratio : Gain  Orientation=left  Gain=-Actuator.GearRatio  SaturateOnIntegerOverflow=on
  Ground : mblibv1/Bodies/Ground  Orientation=left  Opaque=on  LeftPortType=env  RightPortType=workingframe  PhysicalDomain=Mechanical  DialogClass=GroundBlock  CoordPosition=[0 0 0]  CoordPositionUnits=m  StateVectorMgrId=-1  MachineId=[7 1]  ShowEnvPort=on
  Input rotation  freedom : mblibv1/Joints/Revolute  Tag=Factory generic  Description=Mechanical Blockset  Orientation=left  PhysicalDomain=mechanical  SubClassName=Unknown  LeftPortType=blob  RightPortType=blob  LConnTagsString=__newl0|SA1|SA2  RConnTagsString=__newr0|SA1|SA2  NumSAPorts=4  CutJoint=off  MarkAsCut=off  Primitives=revolute  PrimitiveProps=R1$WORLD$Actuator.Axis$revolute  DialogClass=JointBlock
  Integrator : Integrator  Orientation=left  InitialCondition=q0  ZeroCross=off
  Integrator1 : Integrator  Orientation=left  ZeroCross=off
  Joint Actuator : mblibv1/Sensors &  Actuators/Joint Actuator  Orientation=left  Opaque=on  PhysicalDomain=Mechanical  PortType=blob  ActuationStyle=Force  AngleUnits=deg  ArcVelocityUnits=deg/s  ArcAccelerationUnits=deg/s^2  CoordPositionUnits=m  VelocityUnits=m/s  AccelerationUnits=m/s^2  ForceUnits=N  TorqueUnits=N-m  ActiveIO=on  Width=1  DialogClass=MechanicalActuatorBlock  Primitive=R1  ReferenceFrame=Absolute (INERTIAL)
  Joint Initial Condition : mblibv1/Sensors &  Actuators/Joint Initial Condition  Orientation=up  Opaque=on  PhysicalDomain=Mechanical  DialogClass=InitialConditionBlock  Primitive=R1  CoordPosition=q0*Actuator.GearRatio  Velocity=0.0  AngleUnits=rad  ArcVelocityUnits=deg/s  CoordPositionUnits=m  VelocityUnits=m/s  InitialConditions=P1$false$0$m$rad$0$m/s$rad/s#P2$false$0$m$rad$0$m/s$rad/s#P3$false$0$m$rad$0$m/s$rad/s#R1$true$q0*Actuator.GearRatio$m$rad$0.0$m/s$deg/s#R2$false$0$m$rad$0$m/s$rad/s#R3$false$0$m$rad$0$m/s$rad/s#S$false$0$m$rad$0$m/s$rad/s
  Joint Initial Condition1 : mblibv1/Sensors &  Actuators/Joint Initial Condition  Orientation=up  Opaque=on  PhysicalDomain=Mechanical  DialogClass=InitialConditionBlock  Primitive=R1  CoordPosition=q0  Velocity=0.0  AngleUnits=rad  ArcVelocityUnits=deg/s  CoordPositionUnits=m  VelocityUnits=m/s  InitialConditions=P1$false$0$m$rad$0$m/s$rad/s#P2$false$0$m$rad$0$m/s$rad/s#P3$false$0$m$rad$0$m/s$rad/s#R1$true$q0$m$rad$0.0$m/s$deg/s#R2$false$0$m$rad$0$m/s$rad/s#R3$false$0$m$rad$0$m/s$rad/s#S$false$0$m$rad$0$m/s$rad/s
  Machine Environment : mblibv1/Bodies/Mechanical Environment  Tag=Factory ground  Orientation=down  DialogController=MECH.DialogSource  Opaque=on  PortType=env  PhysicalDomain=Mechanical  DialogTemplateClass=MECH.MachineEnvironment  SyncWhenCopied=off  Gravity=[0 -9.81 0]  GravityUnits=m/s^2  GravityAsSignal=off  Dimensionality=3D Only  AnalysisType=Forward dynamics  LinearAssemblyTolerance=1e-3  LinearAssemblyToleranceUnits=m  AngularAssemblyTolerance=1e-3  AngularAssemblyToleranceUnits=rad  ConstraintSolverType=Stabilizing  ConstraintRelTolerance=1e-4  ConstraintAbsTolerance=1e-4  UseRobustSingularityHandling=off  StatePerturbationType=Fixed  PerturbationSize=1e-5  VisualizeMachine=on
  Motor circuitry : Subsystem  Orientation=left  mask{Ri=10, Ra=250, Rd1=100, Rd2=100, Rd3=100, Rd4=100, Rp1=200, Rp2=50, k=Actuator.MotorGain, d=Actuator.MotorDamping, w=Actuator.MotorConstant}
      mask prompts: Ri "Ri (Ohms)"; Ra "Ra (Ohms)"; Rd1 "Rd1 (Ohms)"; Rd2 "Rd2 (Ohms)"; Rd3 "Rd3 (Ohms)"; Rd4 "Rd4 (Ohms)"; Rp1 "Rp1 (Ohms)"; Rp2 "Rp2 (Ohms)"; k "Motor gain (Nm/A)"; d "Motor damping"; w "Motor time constant"
      mask Display: plot(-140,-140,140,140,2*[-30,-30,0,-30,-30,-55]+25,(2*[20,0,20,41,20,20]+8),[0,0]+25,(2*[0,40]+8),2*[37.5,0]+25,(2*[20,20]+8),2*[10,10,0]+25,(1*[-15,6,20]+12),1*[-65,-65,-20,-20,40,40,85,85,85,40,40,-20,-20],1*[48,-20,-20,-10,-10,-20,-20,48,-20,-20,-30,-30,-20])
  Output rotation freedom : mblibv1/Joints/Revolute  Tag=Factory generic  Description=Mechanical Blockset  Orientation=left  PhysicalDomain=mechanical  SubClassName=Unknown  LeftPortType=blob  RightPortType=blob  LConnTagsString=__newl0|SA1|SA2  RConnTagsString=__newr0|SA1  NumSAPorts=3  CutJoint=off  MarkAsCut=off  Primitives=revolute  PrimitiveProps=R1$WORLD$Actuator.Axis$revolute  DialogClass=JointBlock
  Rotor inertia : mblibv1/Bodies/Body  Tag=Factory generic  Description=Mechanical Blockset  Orientation=up  PhysicalDomain=mechanical  SubClassName=Unknown  LeftPortType=workingframe  RightPortType=workingframe  LConnTagsString=CS1  DialogClass=MechanicalBodyBlock  Mass=0  MassUnits=kg  InertiaUnits=kg*m^2  Inertia=Actuator.MotorInertia*eye(3)  Shape=Cylinder  ShapeDims=[1 1]  ShapeUnits=m  ShapeUse=false  Density=1  DensityUnits=kg/m^3  DensityUse=false  CG=Left$CG$[0 0 0]$CS1$CS1$m$[0 0 0]$Euler X-Y-Z$deg$WORLD$false  WorkingFrames=Left$CS1$[0 0 0]$ADJOINING$ADJOINING$m$[0 0 0]$Euler X-Y-Z$deg$WORLD$true
  Shaft stiffnes and damping : Gain  Orientation=left  Gain=[-Actuator.ShaftStiffness -Actuator.ShaftDamping]  Multiplication=Matrix(K*u)  SaturateOnIntegerOverflow=on
  Sum : Sum  Orientation=left  Inputs=-+|  SaturateOnIntegerOverflow=on  InputSameDT=on
  Base : PMIOPort  Tag=PMCPort  Orientation=down  Port=1  Side=Left
  Follower : PMIOPort  Tag=PMCPort  Orientation=down  Port=2  Side=Right
  wires:
  Coulomb friction/1(Angular velocity) -> Controller/1(Angular velocity), Motor circuitry/1(Angular velocity)
  Gear ratio/1 -> Joint Actuator/1  "Drive torque (Nm)"
  Integrator/1 -> Gain4/1
  Acceleration/1 -> Integrator1/1
  "Continuous angle "/1("Out ") -> Sum/1
  Gain2/1 -> Controller/2(w_ref)
  Gain4/1 -> Controller/3(phi_ref)
  Motor circuitry/1(Torque) -> Coulomb friction/1(Motor torque)
  Sum/1 -> Shaft stiffnes and damping/1
  Continuous angle/1(Out) -> Sum/2
  Continuous angle/2(phi) -> Controller/4(phi)
  Shaft stiffnes and damping/1 -> Gear ratio/1, Coulomb friction/2(Gear torque)  "Gear reaction (Nm)"
  Integrator1/1 -> Integrator/1, Gain2/1
  Controller/1(i_ref) -> Motor circuitry/2(i_ref)
  connections:
  Base/RConn1 -- Output rotation freedom/LConn1
  Output rotation freedom/RConn1 -- Follower/RConn1
  Output rotation freedom/RConn2 -- "Continuous angle "/LConn1
  Coulomb friction/RConn1 -- Input rotation  freedom/LConn2
  Coulomb friction/RConn2 -- Input rotation  freedom/LConn3
  Input rotation  freedom/RConn1 -- Rotor inertia/LConn1
  Input rotation  freedom/RConn2 -- Continuous angle/LConn1
  Ground/RConn1 -- Input rotation  freedom/LConn1
  Joint Initial Condition1/RConn1 -- Output rotation freedom/LConn3
  Joint Actuator/RConn1 -- Output rotation freedom/LConn2
  Joint Initial Condition/RConn1 -- Input rotation  freedom/RConn3
  Ground/LConn1 -- Machine Environment/RConn1

== system mech_robot/Robot/Link 2/Subsystem ==
  Clock1 : Clock
      settings: Decimation=10
  Trajectory 2 : Lookup  DialogController=Simulink.DDGSource  InputValues="[0    0.1000    0.1000    1.1000    1.1000    1.2000    1.2000    1.3000]"  OutputValues="[-15   -15     0     0    15    15     0     0]"  SaturateOnIntegerOverflow=on
  Acceleration2 : Outport
  wires:
  Clock1/1 -> Trajectory 2/1
  Trajectory 2/1 -> Acceleration2/1

== system mech_robot/Robot/Link3/Acceleration3 ==
  Clock5 : Clock
      settings: Decimation=10
  Trajectory 3 : Lookup  DialogController=Simulink.DDGSource  InputValues="[0    0.1500    0.1500    0.6000    0.6000    0.9000    0.9000    1.2000    1.2000    1.3000]"  OutputValues="[30.0000   30.0000  -21.5600  -21.5600         0         0   17.3300   17.3300         0         0]"  SaturateOnIntegerOverflow=on
  Acceleration3 : Outport
  wires:
  Clock5/1 -> Trajectory 3/1
  Trajectory 3/1 -> Acceleration3/1

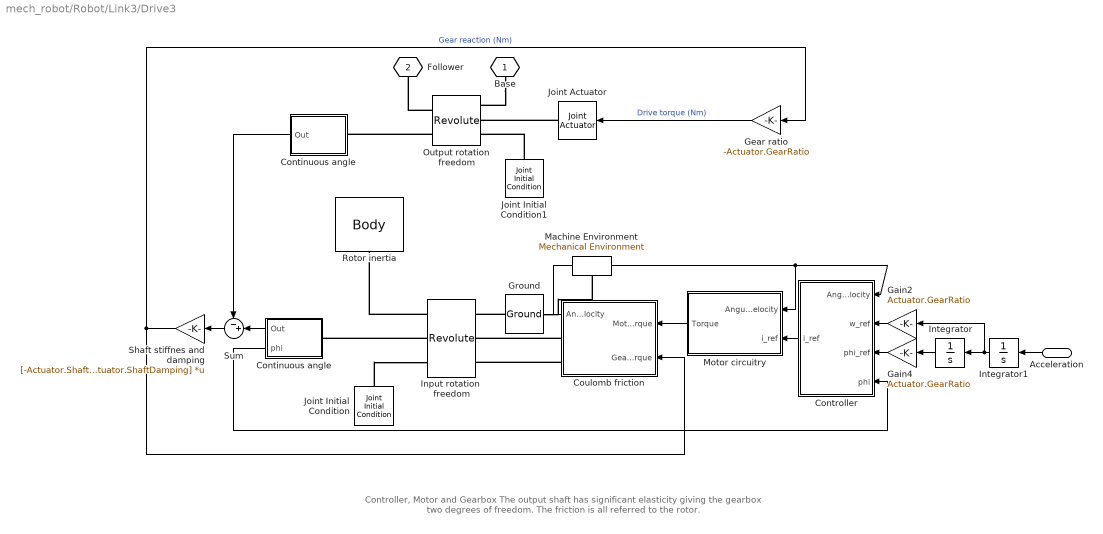
== system mech_robot/Robot/Link3/Drive3 ==
  note: Controller, Motor and Gearbox
      |
      | The output shaft has significant elasticity giving the gearbox two
      | degrees of freedom. The friction is all referred to the rotor.
  Acceleration : Inport  Orientation=left  Port=1  LatchInput=off
  Continuous angle : Subsystem  Orientation=left
  "Continuous angle " : Subsystem  Orientation=left
  Controller : Subsystem  Orientation=left
  Coulomb friction : Subsystem  Orientation=left  mask{peak=Actuator.PeakRatio, Rv1=Actuator.FrictionGain, Rv0=Actuator.FrictionConstant}
      mask prompts: peak "Peak ratio"; Rv1 "Friction gain (Nm.s/rad)"; Rv0 "Friction constant (Nm)"
      mask Display:
      | plot([-2 0 0 2],[-2 -1 1 2]);
      | plot([-5 5],[0 0]);
      | plot([0 0],[-5 5]);
      | plot([-0.02 -0.02],[-3 3]);
      | plot([-0.04 -0.04],[-3 3]);
      | plot([-0.06 -0.06],[-3 3]);
      | plot([-0.08 -0.08],[-3 3]);
      | plot([-0.1 -0.1],[-3 3]);
      | plot([0.02 0.02],[-3 3]);
      | plot([0.04 0.04],[-3 3]);
      | plot([0.06 0.06],[-3 3]);
      | plot([0.08 0.08],[-3 3]);
      | plot([0.1 0.1],[-3 3]);
      | plot([-2 0],[-2.03 -1.03]);
      | plot([-2 0],[-2.06 -1.06]);
      | plot([-2 0],[-2.09 -1.09]);
      | plot([-2 0],[-2.12 -1.21]);
      | plot([-2 0],[-1.97 -0.97]);
      | plot([-2 0],[-1.94 -0.94]);
      | plot([-2 0],[-1.91 -0.91]);
      | plot([-2 0],[-1.88 -0.88]);
      | 
      | plot([2 0],[2.03 1.03]);
      | plot([2 0],[2.06 1.06]);
      | plot([2 0],[2.09 1.09]);
      | plot([2 0],[2.12 1.21]);
      | plot([2 0],[1.97 0.97]);
      | plot([2 0],[1.94 0.94]);
      | plot([2 0],[1.91 0.91]);
      | plot([2 0],[1.88 0.88]);
  Gain2 : Gain  Orientation=left  Gain=Actuator.GearRatio  SaturateOnIntegerOverflow=on
  Gain4 : Gain  Orientation=left  Gain=Actuator.GearRatio  SaturateOnIntegerOverflow=on
  Gear ratio : Gain  Orientation=left  Gain=-Actuator.GearRatio  SaturateOnIntegerOverflow=on
  Ground : mblibv1/Bodies/Ground  Orientation=left  Opaque=on  LeftPortType=env  RightPortType=workingframe  PhysicalDomain=Mechanical  DialogClass=GroundBlock  CoordPosition=[0 0 0]  CoordPositionUnits=m  StateVectorMgrId=-1  MachineId=[7 2]  ShowEnvPort=on
  Input rotation  freedom : mblibv1/Joints/Revolute  Tag=Factory generic  Description=Mechanical Blockset  Orientation=left  PhysicalDomain=mechanical  SubClassName=Unknown  LeftPortType=blob  RightPortType=blob  LConnTagsString=__newl0|SA1|SA2  RConnTagsString=__newr0|SA1|SA2  NumSAPorts=4  CutJoint=off  MarkAsCut=off  Primitives=revolute  PrimitiveProps=R1$WORLD$Actuator.Axis$revolute  DialogClass=JointBlock
  Integrator : Integrator  Orientation=left  InitialCondition=q0  ZeroCross=off
  Integrator1 : Integrator  Orientation=left  ZeroCross=off
  Joint Actuator : mblibv1/Sensors &  Actuators/Joint Actuator  Orientation=left  Opaque=on  PhysicalDomain=Mechanical  PortType=blob  ActuationStyle=Force  AngleUnits=deg  ArcVelocityUnits=deg/s  ArcAccelerationUnits=deg/s^2  CoordPositionUnits=m  VelocityUnits=m/s  AccelerationUnits=m/s^2  ForceUnits=N  TorqueUnits=N-m  ActiveIO=on  Width=1  DialogClass=MechanicalActuatorBlock  Primitive=R1  ReferenceFrame=Absolute (INERTIAL)
  Joint Initial Condition : mblibv1/Sensors &  Actuators/Joint Initial Condition  Orientation=up  Opaque=on  PhysicalDomain=Mechanical  DialogClass=InitialConditionBlock  Primitive=R1  CoordPosition=q0*Actuator.GearRatio  Velocity=0.0  AngleUnits=rad  ArcVelocityUnits=deg/s  CoordPositionUnits=m  VelocityUnits=m/s  InitialConditions=P1$false$0$m$rad$0$m/s$rad/s#P2$false$0$m$rad$0$m/s$rad/s#P3$false$0$m$rad$0$m/s$rad/s#R1$true$q0*Actuator.GearRatio$m$rad$0.0$m/s$deg/s#R2$false$0$m$rad$0$m/s$rad/s#R3$false$0$m$rad$0$m/s$rad/s#S$false$0$m$rad$0$m/s$rad/s
  Joint Initial Condition1 : mblibv1/Sensors &  Actuators/Joint Initial Condition  Orientation=up  Opaque=on  PhysicalDomain=Mechanical  DialogClass=InitialConditionBlock  Primitive=R1  CoordPosition=q0  Velocity=0.0  AngleUnits=rad  ArcVelocityUnits=deg/s  CoordPositionUnits=m  VelocityUnits=m/s  InitialConditions=P1$false$0$m$rad$0$m/s$rad/s#P2$false$0$m$rad$0$m/s$rad/s#P3$false$0$m$rad$0$m/s$rad/s#R1$true$q0$m$rad$0.0$m/s$deg/s#R2$false$0$m$rad$0$m/s$rad/s#R3$false$0$m$rad$0$m/s$rad/s#S$false$0$m$rad$0$m/s$rad/s
  Machine Environment : mblibv1/Bodies/Mechanical Environment  Tag=Factory ground  Orientation=down  DialogController=MECH.DialogSource  Opaque=on  PortType=env  PhysicalDomain=Mechanical  DialogTemplateClass=MECH.MachineEnvironment  SyncWhenCopied=off  Gravity=[0 -9.81 0]  GravityUnits=m/s^2  GravityAsSignal=off  Dimensionality=3D Only  AnalysisType=Forward dynamics  LinearAssemblyTolerance=1e-3  LinearAssemblyToleranceUnits=m  AngularAssemblyTolerance=1e-3  AngularAssemblyToleranceUnits=rad  ConstraintSolverType=Stabilizing  ConstraintRelTolerance=1e-4  ConstraintAbsTolerance=1e-4  UseRobustSingularityHandling=off  StatePerturbationType=Fixed  PerturbationSize=1e-5  VisualizeMachine=on
  Motor circuitry : Subsystem  Orientation=left  mask{Ri=10, Ra=250, Rd1=100, Rd2=100, Rd3=100, Rd4=100, Rp1=200, Rp2=50, k=Actuator.MotorGain, d=Actuator.MotorDamping, w=Actuator.MotorConstant}
      mask prompts: Ri "Ri (Ohms)"; Ra "Ra (Ohms)"; Rd1 "Rd1 (Ohms)"; Rd2 "Rd2 (Ohms)"; Rd3 "Rd3 (Ohms)"; Rd4 "Rd4 (Ohms)"; Rp1 "Rp1 (Ohms)"; Rp2 "Rp2 (Ohms)"; k "Motor gain (Nm/A)"; d "Motor damping"; w "Motor time constant"
      mask Display: plot(-140,-140,140,140,2*[-30,-30,0,-30,-30,-55]+25,(2*[20,0,20,41,20,20]+8),[0,0]+25,(2*[0,40]+8),2*[37.5,0]+25,(2*[20,20]+8),2*[10,10,0]+25,(1*[-15,6,20]+12),1*[-65,-65,-20,-20,40,40,85,85,85,40,40,-20,-20],1*[48,-20,-20,-10,-10,-20,-20,48,-20,-20,-30,-30,-20])
  Output rotation freedom : mblibv1/Joints/Revolute  Tag=Factory generic  Description=Mechanical Blockset  Orientation=left  PhysicalDomain=mechanical  SubClassName=Unknown  LeftPortType=blob  RightPortType=blob  LConnTagsString=__newl0|SA1|SA2  RConnTagsString=__newr0|SA1  NumSAPorts=3  CutJoint=off  MarkAsCut=off  Primitives=revolute  PrimitiveProps=R1$WORLD$Actuator.Axis$revolute  DialogClass=JointBlock
  Rotor inertia : mblibv1/Bodies/Body  Tag=Factory generic  Description=Mechanical Blockset  Orientation=up  PhysicalDomain=mechanical  SubClassName=Unknown  LeftPortType=workingframe  RightPortType=workingframe  LConnTagsString=CS1  DialogClass=MechanicalBodyBlock  Mass=0  MassUnits=kg  InertiaUnits=kg*m^2  Inertia=Actuator.MotorInertia*eye(3)  Shape=Cylinder  ShapeDims=[1 1]  ShapeUnits=m  ShapeUse=false  Density=1  DensityUnits=kg/m^3  DensityUse=false  CG=Left$CG$[0 0 0]$CS1$CS1$m$[0 0 0]$Euler X-Y-Z$deg$WORLD$false  WorkingFrames=Left$CS1$[0 0 0]$ADJOINING$ADJOINING$m$[0 0 0]$Euler X-Y-Z$deg$WORLD$true
  Shaft stiffnes and damping : Gain  Orientation=left  Gain=[-Actuator.ShaftStiffness -Actuator.ShaftDamping]  Multiplication=Matrix(K*u)  SaturateOnIntegerOverflow=on
  Sum : Sum  Orientation=left  Inputs=-+|  SaturateOnIntegerOverflow=on  InputSameDT=on
  Base : PMIOPort  Tag=PMCPort  Orientation=down  Port=1  Side=Left
  Follower : PMIOPort  Tag=PMCPort  Orientation=down  Port=2  Side=Right
  wires:
  Coulomb friction/1(Angular velocity) -> Controller/1(Angular velocity), Motor circuitry/1(Angular velocity)
  Gear ratio/1 -> Joint Actuator/1  "Drive torque (Nm)"
  Integrator/1 -> Gain4/1
  Acceleration/1 -> Integrator1/1
  "Continuous angle "/1("Out ") -> Sum/1
  Gain2/1 -> Controller/2(w_ref)
  Gain4/1 -> Controller/3(phi_ref)
  Controller/1(i_ref) -> Motor circuitry/2(i_ref)
  Motor circuitry/1(Torque) -> Coulomb friction/1(Motor torque)
  Sum/1 -> Shaft stiffnes and damping/1
  Continuous angle/1(Out) -> Sum/2
  Continuous angle/2(phi) -> Controller/4(phi)
  Integrator1/1 -> Integrator/1, Gain2/1
  Shaft stiffnes and damping/1 -> Gear ratio/1, Coulomb friction/2(Gear torque)  "Gear reaction (Nm)"
  connections:
  Base/RConn1 -- Output rotation freedom/LConn1
  Output rotation freedom/RConn1 -- Follower/RConn1
  Output rotation freedom/RConn2 -- "Continuous angle "/LConn1
  Coulomb friction/RConn1 -- Input rotation  freedom/LConn2
  Coulomb friction/RConn2 -- Input rotation  freedom/LConn3
  Input rotation  freedom/RConn1 -- Rotor inertia/LConn1
  Input rotation  freedom/RConn2 -- Continuous angle/LConn1
  Ground/RConn1 -- Input rotation  freedom/LConn1
  Joint Initial Condition1/RConn1 -- Output rotation freedom/LConn3
  Joint Actuator/RConn1 -- Output rotation freedom/LConn2
  Joint Initial Condition/RConn1 -- Input rotation  freedom/RConn3
  Ground/LConn1 -- Machine Environment/RConn1
